simulink model "a_1_Schema_di_controllo"  (R2019a)
settings: Solver=VariableStepAuto  StartTime=0.0  StopTime=100  RelTol=1e-3
libraries: cstblocks x2
settings Model: Creator=Samuele  LastModifiedBy=Samuele

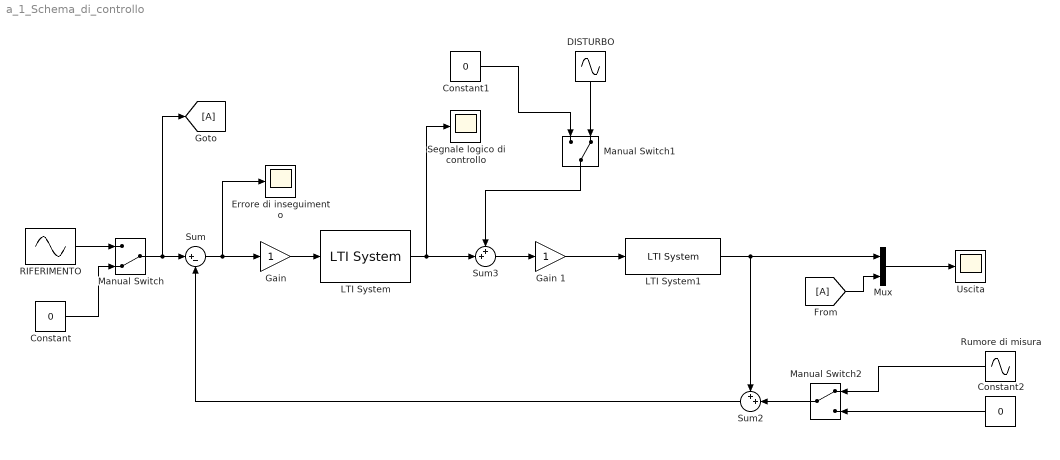
== system a_1_Schema_di_controllo ==
  Constant : Constant  Value=0
  Constant1 : Constant  Value=0
  Constant2 : Constant  Value=0
  "DISTURBO " : Sin  Frequency=1/40  SampleTime=0
  Errore di inseguimento : Scope
  Gain : Gain
  Gain 1 : Gain
  LTI System : cstblocks/LTI System  sys=C  IC=[]
  LTI System1 : cstblocks/LTI System  sys=G  IC=[]
  Manual Switch : ManualSwitch  CurrentSetting=0
  Manual Switch1 : ManualSwitch  CurrentSetting=0
  Manual Switch2 : ManualSwitch
  Mux : Mux  Inputs=2
  "RIFERIMENTO " : Sin  Frequency=1/5  SampleTime=0
  Rumore di misura : Sin  Frequency=60  SampleTime=0
  Segnale logico di controllo : Scope
  Sum : Sum  Inputs=|+-
  Sum2 : Sum  Inputs=++|
  Sum3 : Sum  Inputs=++|
  Uscita : Scope
  wires:
  Sum/1 -> Gain/1, Errore di inseguimento/1
  Gain/1 -> LTI System/1
  Gain 1/1 -> LTI System1/1
  Manual Switch/1 -> [A], Sum/1
  Constant/1 -> Manual Switch/2
  "RIFERIMENTO "/1 -> Manual Switch/1
  LTI System/1 -> Sum3/2, Segnale logico di controllo/1
  Sum3/1 -> Gain 1/1
  Manual Switch1/1 -> Sum3/1
  "DISTURBO "/1 -> Manual Switch1/2
  Constant1/1 -> Manual Switch1/1
  Sum2/1 -> Sum/2
  Rumore di misura/1 -> Manual Switch2/1
  Constant2/1 -> Manual Switch2/2
  Manual Switch2/1 -> Sum2/2
  Mux/1 -> Uscita/1
  LTI System1/1 -> Sum2/1, Mux/1
  [A] -> Mux/2
